simulink subsystem "slip_model"  (R2024b)
settings: Solver=VariableStepAuto  StartTime=0.0  StopTime=10.0  RelTol=1e-3
model mask{radius=0, min_velocity=0}
  mask prompts: radius "Radius [m]"; min_velocity "Minimum velocity [m/s]"
settings Model: Creator=yevge  LastModifiedBy=yevge

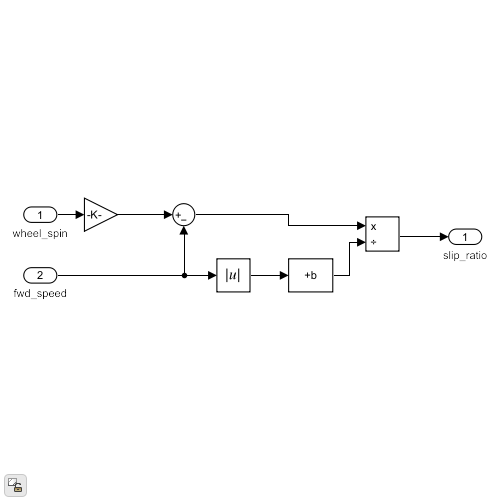
[thumbnail: Simulink's stored preview of the top-level diagram]
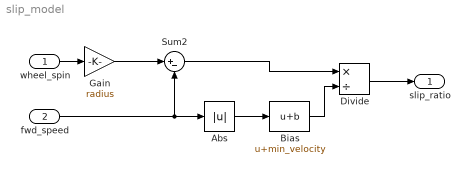
== system slip_model ==
  wheel_spin : Inport  Unit=rad/s
  fwd_speed : Inport  Port=2  Unit=m/s
  Abs : Abs  SaturateOnIntegerOverflow=off
  Bias : Bias  Bias=min_velocity  SaturateOnIntegerOverflow=off
  Divide : Product  Inputs=*/
  Gain : Gain  Gain=radius
  Sum2 : Sum  Inputs=|+-
  slip_ratio : Outport  Unit=1
  wires:
  Abs/1 -> Bias/1
  Sum2/1 -> Divide/1
  Bias/1 -> Divide/2
  fwd_speed/1 -> Abs/1, Sum2/2
  Gain/1 -> Sum2/1
  Divide/1 -> slip_ratio/1
  wheel_spin/1 -> Gain/1
